simulink model "lab5_3"  (R2018a)
settings: Solver=VariableStepAuto  StartTime=0.0  StopTime=20  MaxStep=0.001  RelTol=1e-3
libraries: powerlib x4, ECEN315_Library x2, ECEN315_Library_Fault x1
settings Model: Creator=joshua  LastModifiedBy=joshua

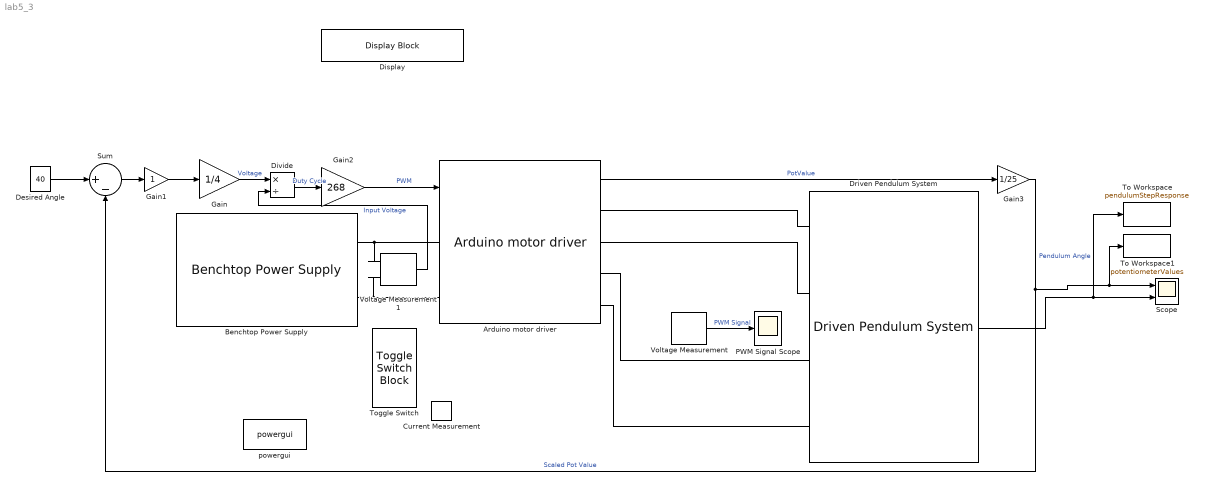
== system lab5_3 ==
  Arduino motor driver : ECEN315_Library_Fault/Arduino motor driver  E=off
  Benchtop Power Supply : ECEN315_Library/Benchtop Power Supply  V=12
  Current Measurement : powerlib/Measurements/Current Measurement  PhasorSimulation=off  OutputType=Complex  PSBequivalent=0
  Desired Angle : Constant  Value=40  VectorParams1D=off  OutDataTypeStr=double
  Display : DisplayBlock  WebBlockId=38  LabelPosition=Hide
  Divide : Product  Inputs=*/
  Driven Pendulum System : ECEN315_Library/Driven Pendulum System  SystemSampleTime=-1
  Gain : Gain  Gain=1/4
  Gain1 : Gain
  Gain2 : Gain  Gain=268
  Gain3 : Gain  Gain=1/25
  PWM Signal Scope : Scope
  Scope : Scope  NumInputPorts=2
  Sum : Sum  Inputs=|+-
  To Workspace : ToWorkspace  VariableName=pendulumStepResponse  SampleTime=-1
      settings: Save2DSignal=2-D array (concatenate along first dimension)
  To Workspace1 : ToWorkspace  VariableName=potentiometerValues  SampleTime=-1
      settings: Save2DSignal=2-D array (concatenate along first dimension)
  Toggle Switch : ToggleSwitchBlock  WebBlockId=55
      settings: Values={{'Off', 'On'}, [0 12]}
  Voltage Measurement : powerlib/Measurements/Voltage Measurement  PhasorSimulation=off  OutputType=Complex  PSBequivalent=0
  Voltage Measurement1 : powerlib/Measurements/Voltage Measurement  PhasorSimulation=off  OutputType=Complex  PSBequivalent=0
  powergui : powerlib/powergui  Priority=1  SimulationMode=Continuous  SampleTime=50e-6  frequency=60  Iterations=50  frequencyindice=0  Pbase=100e6  ErrMax=1e-4  UnitsV=kV  UnitsW=MW  buscounter=0  FunctionMessages=off  echomessages=off  EnableUseOfTLC=off  CurrentSourceSwitches=off  DisableSnubberDevices=off  DisableRonSwitches=off  DisableVfSwitches=off  DisplayEquations=off  SolverType=Tustin/Backward Euler (TBE)  Interpol=off  ExternalGateDelay=off  methode=off  Ts=100  x0status=blocks  SPID=on  SwTol=0  HookPort=off  RestoreLinks=warning  ResistiveCurrentMeasurement=off  Frange=[0:2:500]  Ylog=off  Xlog=on  ShowGrid=off  save=off  variable=ZData  structure=0  ZoomFFT=off  StartTime=0.0  cycles=1  DisplayStyle=1  fundamental=60  FreqAxis=off  MaxFrequency=1000  frequencyindicesteady=1  RmsSteady=1  display=off
  wires:
  Driven Pendulum System/1 -> To Workspace/1, Scope/2  "Pendulum Angle"
  Gain3/1 -> To Workspace1/1, Scope/1, Sum/2  "Scaled Pot Value"
  Arduino motor driver/1 -> Gain3/1  "PotValue"
  Voltage Measurement/1 -> PWM Signal Scope/1  "PWM Signal"
  Voltage Measurement1/1 -> Divide/2  "Input Voltage"
  Divide/1 -> Gain2/1  "Duty Cycle"
  Gain/1 -> Divide/1  "Voltage"
  Desired Angle/1 -> Sum/1
  Gain2/1 -> Arduino motor driver/1  "PWM"
  Sum/1 -> Gain1/1
  Gain1/1 -> Gain/1
  connections:
  Arduino motor driver/RConn1 -- Driven Pendulum System/LConn1
  Arduino motor driver/RConn2 -- Driven Pendulum System/LConn2
  Arduino motor driver/LConn1 -- Voltage Measurement1/LConn1 -- Benchtop Power Supply/RConn1
  Benchtop Power Supply/RConn2 -- Voltage Measurement1/LConn2 -- Arduino motor driver/LConn2
  Driven Pendulum System/LConn3 -- Arduino motor driver/RConn3
  Driven Pendulum System/LConn4 -- Arduino motor driver/RConn4
